simulink model "ball_nozerocross"  (Simulink 9.0)
settings: Solver=ode45  StartTime=0.0  StopTime=7  RelTol=1e-2  EnableMultiTasking=on
settings Model: Creator=Knut  LastModifiedBy=Knut
settings SolverCC: ZeroCrossControl=DisableAll
settings DataIOCC: LimitDataPoints=on  SignalLoggingSaveFormat=ModelDataLogs
settings OptimizationCC: BlockReduction=off  BooleanDataType=off  LifeSpan=auto
settings DebuggingCC: SaveWithParameterizedLinksMsg=none  SignalResolutionControl=TryResolveAllWithWarning  MultiTaskDSMMsg=warning  MultiTaskCondExecSysMsg=none  SFUnexpectedBacktrackingDiag=error  SFNoUnconditionalDefaultTransitionDiag=error  SFExecutionAtInitializationDiag=warning
settings HardwareCC: ProdBitPerPointer=64  ProdBitPerSizeT=64  ProdBitPerPtrDiffT=64  ProdLargestAtomicFloat=Float  ProdIntDivRoundTo=Zero  ProdEndianess=LittleEndian  ProdWordSize=64  ProdHWDeviceType=Intel->x86-64 (Windows64)  TargetUnknown=on
settings GRTTargetCC: CombineOutputUpdateFcns=off  GRTInterface=on
settings ConfigComp: CovMetricSettings=dwe

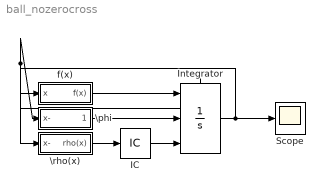
== system ball_nozerocross ==
  IC : InitialCondition  Value=[10;5]
  Integrator : Integrator  ExternalReset=rising  InitialConditionSource=external  ShowStatePort=on
  Scope : Scope
  \phi : Subsystem  Description=f(x)
  \rho(x) : Subsystem  Description=f(x)
  f(x) : Subsystem  Description=f(x)
  wires:
  IC/1 -> Integrator/3
  f(x)/1(f(x)) -> Integrator/1
  \phi/1(x\in\phi) -> Integrator/2
  Integrator/State -> \rho(x)/1(x-), \phi/1(x-)
  \rho(x)/1(rho(x)) -> IC/1
  Integrator/1 -> f(x)/1(x), Scope/1

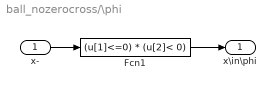
== system ball_nozerocross/\phi ==
  x- : Inport
  Fcn1 : Fcn  Expr=(u[1]<=0) * (u[2]< 0)
  x\in\phi : Outport
  wires:
  x-/1 -> Fcn1/1
  Fcn1/1 -> x\in\phi/1

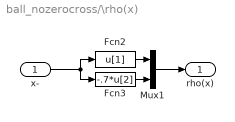
== system ball_nozerocross/\rho(x) ==
  x- : Inport
  Fcn2 : Fcn  Expr=u[1]
  Fcn3 : Fcn  Expr=-.7*u[2]
  Mux1 : Mux  Inputs=2
  rho(x) : Outport
  wires:
  Fcn3/1 -> Mux1/2
  Fcn2/1 -> Mux1/1
  Mux1/1 -> rho(x)/1
  x-/1 -> Fcn2/1, Fcn3/1

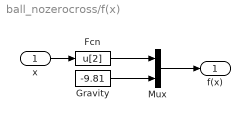
== system ball_nozerocross/f(x) ==
  x : Inport
  Fcn : Fcn  Expr=u[2]
  Gravity : Constant  Value=-9.81
  Mux : Mux  Inputs=2
  f(x) : Outport
  wires:
  Mux/1 -> f(x)/1
  Gravity/1 -> Mux/2
  Fcn/1 -> Mux/1
  x/1 -> Fcn/1
